simulink model "q2c"  (R2017a)
settings: Solver=VariableStepAuto  StartTime=0.0  StopTime=10.0  RelTol=1e-3
settings Model: Creator=adamhzp  LastModifiedBy=adamhzp

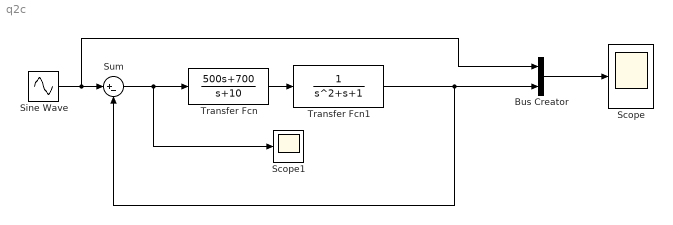
== system q2c ==
  Bus Creator : BusCreator  Inputs=2
  Scope : Scope
  Scope1 : Scope
  Sine Wave : Sin  SampleTime=0
  Sum : Sum  Inputs=|+-
  Transfer Fcn : TransferFcn  Numerator=[500 700]  Denominator=[1 10]
  Transfer Fcn1 : TransferFcn  Denominator=[1 1 1]
  wires:
  Transfer Fcn/1 -> Transfer Fcn1/1
  Sine Wave/1 -> Bus Creator/1, Sum/1
  Bus Creator/1 -> Scope/1
  Sum/1 -> Scope1/1, Transfer Fcn/1
  Transfer Fcn1/1 -> Sum/2, Bus Creator/2
